simulink model "crs_controller"  (R2020b)
settings: Solver=FixedStepDiscrete  StartTime=0.0  StopTime=10.0  FixedStep=Ts  RelTol=1e-3
settings Model: DataDictionary=crs_controllerdic.sldd  EnableAccessToBaseWorkspace=off  Creator=The MathWorks, Inc.  LastModifiedBy=jpulipat
settings DataIOCC: SaveOutput=off  SignalLogging=off  DSMLogging=off  SaveTime=off  ReturnWorkspaceOutputs=off
settings OptimizationCC: DefaultParameterBehavior=Inlined  PassReuseOutputArgsAs=Individual arguments  EfficientTunableParamExpr=on
settings DebuggingCC: ParameterTunabilityLossMsg=error  ArithmeticOperatorsInVariantConditions=warning
settings SFSimCC: SimUseLocalCustomCode=off  CustomCodeUndefinedFunction=UseInterfaceOnly
settings RTWCC: Description=Embedded Coder  SystemTargetFile=ert.tlc  GenCodeOnly=on  TemplateMakefile=ert_default_tmf  GenerateReport=on  RTWUseLocalCustomCode=off  IncludeHyperlinkInReport=on  LaunchReport=on  GenerateTraceInfo=on  GenerateTraceReport=on  GenerateTraceReportSl=on  GenerateTraceReportSf=on  GenerateTraceReportEml=on
settings CodeAppCC: ForceParamTrailComments=on  IgnoreCustomStorageClasses=off  OperatorAnnotations=on  SimulinkDataObjDesc=on  SFDataObjDesc=on  MATLABFcnDesc=on  InsertBlockDesc=on  StateflowObjectComments=on  MATLABSourceComments=on  ReqsInCode=on
settings ERTTargetCC: TargetLangStandard=C99 (ISO)  GenerateSampleERTMain=on  InlinedParameterPlacement=NonHierarchical  ERTCustomFileTemplate=example_file_process.tlc

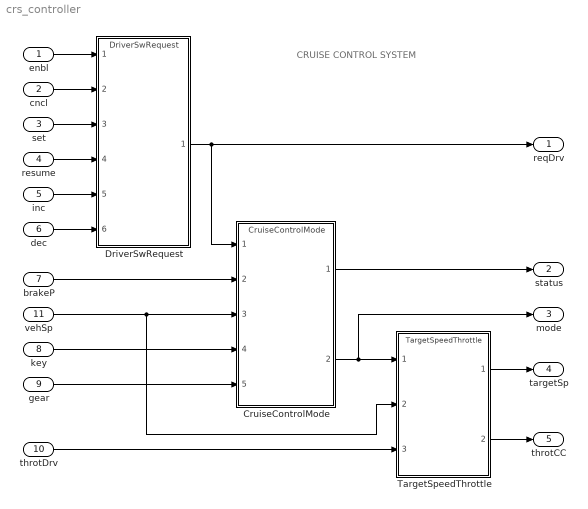
== system crs_controller ==
  note: CRUISE CONTROL SYSTEM
  enbl : Inport  OutDataTypeStr=boolean
  cncl : Inport  Port=2  OutDataTypeStr=boolean
  set : Inport  Port=3  OutDataTypeStr=boolean
  resume : Inport  Port=4  OutDataTypeStr=boolean
  inc : Inport  Port=5  OutDataTypeStr=boolean
  dec : Inport  Port=6  OutDataTypeStr=boolean
  brakeP : Inport  Port=7
  key : Inport  Port=8
  gear : Inport  Port=9  Interpolate=off
  throtDrv : Inport  Port=10
  vehSp : Inport  Port=11
  CruiseControlMode : ModelReference  ModelNameDialog=CruiseControlMode.slx  SimulationMode=Normal  ModelReferenceVersion=4.7
  DriverSwRequest : ModelReference  ModelNameDialog=DriverSwRequest  SimulationMode=Normal  ModelReferenceVersion=4.8
  TargetSpeedThrottle : ModelReference  ModelNameDialog=TargetSpeedThrottle  SimulationMode=Normal  ModelReferenceVersion=4.7
  reqDrv : Outport  VectorParamsAs1DForOutWhenUnconnected=off
  status : Outport  Port=2  VectorParamsAs1DForOutWhenUnconnected=off
  mode : Outport  Port=3  VectorParamsAs1DForOutWhenUnconnected=off
  targetSp : Outport  Port=4  VectorParamsAs1DForOutWhenUnconnected=off
  throtCC : Outport  Port=5  VectorParamsAs1DForOutWhenUnconnected=off
  wires:
  dec/1 -> DriverSwRequest/6
  inc/1 -> DriverSwRequest/5
  enbl/1 -> DriverSwRequest/1
  vehSp/1 -> TargetSpeedThrottle/2, CruiseControlMode/3
  CruiseControlMode/2 -> mode/1, TargetSpeedThrottle/1
  throtDrv/1 -> TargetSpeedThrottle/3
  TargetSpeedThrottle/2 -> throtCC/1
  DriverSwRequest/1 -> reqDrv/1, CruiseControlMode/1
  resume/1 -> DriverSwRequest/4
  set/1 -> DriverSwRequest/3
  CruiseControlMode/1 -> status/1
  TargetSpeedThrottle/1 -> targetSp/1
  gear/1 -> CruiseControlMode/5
  cncl/1 -> DriverSwRequest/2
  brakeP/1 -> CruiseControlMode/2
  key/1 -> CruiseControlMode/4
